simulink model "Com_ISE"  (R2016a)
settings: Solver=VariableStepAuto  StartTime=0.0  StopTime=120  RelTol=1e-3
libraries: simulink x4
settings Model: Creator=Admin  LastModifiedBy=Admin

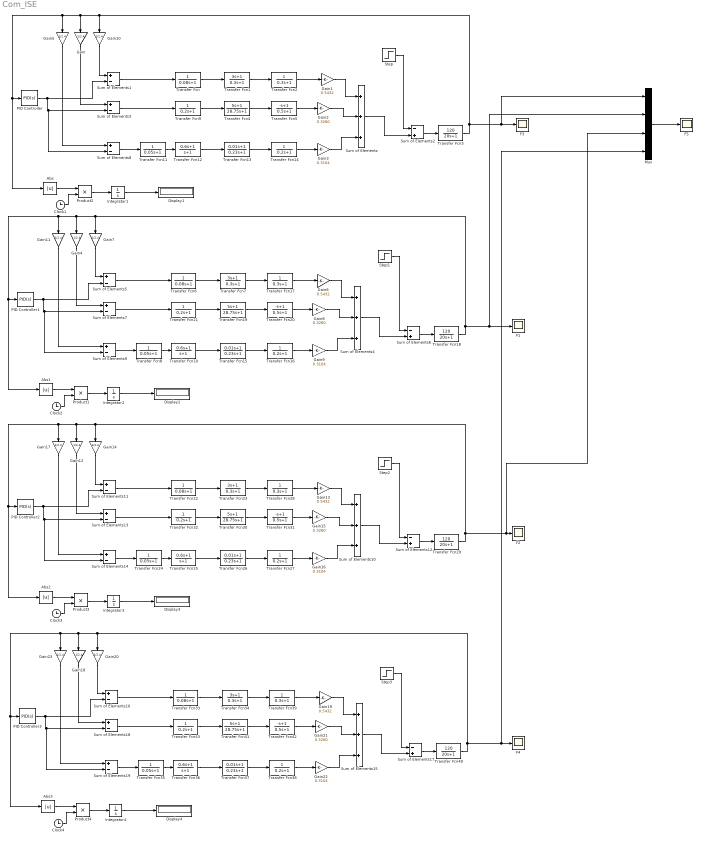
== system Com_ISE ==
  Abs{,1..3} (4 alike) : Abs
  Clock{1..4} (4 alike) : Clock
  Display{1..4} (4 alike) : Display
  F{1..5} (5 alike) : Scope
  Gain{,4..5,7,10..12,14,17..18,20,23} (12 alike) : Gain  Gain=1/2.4
  Gain{1,6,13,19} (4 alike) : Gain  Gain=0.5432
  Gain{2,8,15,21} (4 alike) : Gain  Gain=0.3260
  Gain{3,9,16,22} (4 alike) : Gain  Gain=0.3104
  Integrator{1..4} (4 alike) : Integrator
  Mux : Mux
  PID Controller : simulink/Continuous/PID Controller  Controller=PID  TimeDomain=Continuous-time  SampleTime=-1  IntegratorMethod=Forward Euler  FilterMethod=Forward Euler  Form=Parallel  UseFilter=on  ControllerParametersSource=internal  P=1.2  I=0.4  D=0.11  N=100  InitialConditionSource=internal  InitialConditionForIntegrator=0  InitialConditionForFilter=0  ExternalReset=none  LimitOutput=off  UpperSaturationLimit=inf  LowerSaturationLimit=-inf  LinearizeAsGain=on  AntiWindupMode=none  Kb=1  TrackingMode=off  Kt=1  PParamMin=[]  PParamMax=[]  IParamMin=[]  IParamMax=[]  DParamMin=[]  DParamMax=[]  NParamMin=[]  NParamMax=[]  KbParamMin=[]  KbParamMax=[]  KtParamMin=[]  KtParamMax=[]  POutMin=[]  POutMax=[]  IOutMin=[]  IOutMax=[]  DOutMin=[]  DOutMax=[]  NOutMin=[]  NOutMax=[]  KbOutMin=[]  KbOutMax=[]  KtOutMin=[]  KtOutMax=[]  IntegratorOutMin=[]  IntegratorOutMax=[]  FilterOutMin=[]  FilterOutMax=[]  SumOutMin=[]  SumOutMax=[]  SumI1OutMin=[]  SumI1OutMax=[]  SumI2OutMin=[]  SumI2OutMax=[]  SumI3OutMin=[]  SumI3OutMax=[]  SumDOutMin=[]  SumDOutMax=[]  SaturationOutMin=[]  SaturationOutMax=[]  IntegratorContinuousStateAttributes=''  IntegratorStateMustResolveToSignalObject=off  IntegratorRTWStateStorageClass=Auto  FilterContinuousStateAttributes=''  FilterStateMustResolveToSignalObject=off  FilterRTWStateStorageClass=Auto  DifferentiatorICPrevScaledInput=0  DifferentiatorOutMin=[]  DifferentiatorOutMax=[]
  PID Controller1 : simulink/Continuous/PID Controller  Controller=PID  TimeDomain=Continuous-time  SampleTime=-1  IntegratorMethod=Forward Euler  FilterMethod=Forward Euler  Form=Parallel  UseFilter=on  ControllerParametersSource=internal  P=0.985192773  I=0.993117653  D=0.130440892  N=100  InitialConditionSource=internal  InitialConditionForIntegrator=0  InitialConditionForFilter=0  ExternalReset=none  LimitOutput=off  UpperSaturationLimit=inf  LowerSaturationLimit=-inf  LinearizeAsGain=on  AntiWindupMode=none  Kb=1  TrackingMode=off  Kt=1  PParamMin=[]  PParamMax=[]  IParamMin=[]  IParamMax=[]  DParamMin=[]  DParamMax=[]  NParamMin=[]  NParamMax=[]  KbParamMin=[]  KbParamMax=[]  KtParamMin=[]  KtParamMax=[]  POutMin=[]  POutMax=[]  IOutMin=[]  IOutMax=[]  DOutMin=[]  DOutMax=[]  NOutMin=[]  NOutMax=[]  KbOutMin=[]  KbOutMax=[]  KtOutMin=[]  KtOutMax=[]  IntegratorOutMin=[]  IntegratorOutMax=[]  FilterOutMin=[]  FilterOutMax=[]  SumOutMin=[]  SumOutMax=[]  SumI1OutMin=[]  SumI1OutMax=[]  SumI2OutMin=[]  SumI2OutMax=[]  SumI3OutMin=[]  SumI3OutMax=[]  SumDOutMin=[]  SumDOutMax=[]  SaturationOutMin=[]  SaturationOutMax=[]  IntegratorContinuousStateAttributes=''  IntegratorStateMustResolveToSignalObject=off  IntegratorRTWStateStorageClass=Auto  FilterContinuousStateAttributes=''  FilterStateMustResolveToSignalObject=off  FilterRTWStateStorageClass=Auto  DifferentiatorICPrevScaledInput=0  DifferentiatorOutMin=[]  DifferentiatorOutMax=[]
  PID Controller2 : simulink/Continuous/PID Controller  Controller=PID  TimeDomain=Continuous-time  SampleTime=-1  IntegratorMethod=Forward Euler  FilterMethod=Forward Euler  Form=Parallel  UseFilter=on  ControllerParametersSource=internal  P=0.9999  I=0.9999  D=0.170426245  N=100  InitialConditionSource=internal  InitialConditionForIntegrator=0  InitialConditionForFilter=0  ExternalReset=none  LimitOutput=off  UpperSaturationLimit=inf  LowerSaturationLimit=-inf  LinearizeAsGain=on  AntiWindupMode=none  Kb=1  TrackingMode=off  Kt=1  PParamMin=[]  PParamMax=[]  IParamMin=[]  IParamMax=[]  DParamMin=[]  DParamMax=[]  NParamMin=[]  NParamMax=[]  KbParamMin=[]  KbParamMax=[]  KtParamMin=[]  KtParamMax=[]  POutMin=[]  POutMax=[]  IOutMin=[]  IOutMax=[]  DOutMin=[]  DOutMax=[]  NOutMin=[]  NOutMax=[]  KbOutMin=[]  KbOutMax=[]  KtOutMin=[]  KtOutMax=[]  IntegratorOutMin=[]  IntegratorOutMax=[]  FilterOutMin=[]  FilterOutMax=[]  SumOutMin=[]  SumOutMax=[]  SumI1OutMin=[]  SumI1OutMax=[]  SumI2OutMin=[]  SumI2OutMax=[]  SumI3OutMin=[]  SumI3OutMax=[]  SumDOutMin=[]  SumDOutMax=[]  SaturationOutMin=[]  SaturationOutMax=[]  IntegratorContinuousStateAttributes=''  IntegratorStateMustResolveToSignalObject=off  IntegratorRTWStateStorageClass=Auto  FilterContinuousStateAttributes=''  FilterStateMustResolveToSignalObject=off  FilterRTWStateStorageClass=Auto  DifferentiatorICPrevScaledInput=0  DifferentiatorOutMin=[]  DifferentiatorOutMax=[]
  PID Controller3 : simulink/Continuous/PID Controller  Controller=PID  TimeDomain=Continuous-time  SampleTime=-1  IntegratorMethod=Forward Euler  FilterMethod=Forward Euler  Form=Parallel  UseFilter=on  ControllerParametersSource=internal  P=0.996752419  I=0.999717196  D=0.131550881  N=100  InitialConditionSource=internal  InitialConditionForIntegrator=0  InitialConditionForFilter=0  ExternalReset=none  LimitOutput=off  UpperSaturationLimit=inf  LowerSaturationLimit=-inf  LinearizeAsGain=on  AntiWindupMode=none  Kb=1  TrackingMode=off  Kt=1  PParamMin=[]  PParamMax=[]  IParamMin=[]  IParamMax=[]  DParamMin=[]  DParamMax=[]  NParamMin=[]  NParamMax=[]  KbParamMin=[]  KbParamMax=[]  KtParamMin=[]  KtParamMax=[]  POutMin=[]  POutMax=[]  IOutMin=[]  IOutMax=[]  DOutMin=[]  DOutMax=[]  NOutMin=[]  NOutMax=[]  KbOutMin=[]  KbOutMax=[]  KtOutMin=[]  KtOutMax=[]  IntegratorOutMin=[]  IntegratorOutMax=[]  FilterOutMin=[]  FilterOutMax=[]  SumOutMin=[]  SumOutMax=[]  SumI1OutMin=[]  SumI1OutMax=[]  SumI2OutMin=[]  SumI2OutMax=[]  SumI3OutMin=[]  SumI3OutMax=[]  SumDOutMin=[]  SumDOutMax=[]  SaturationOutMin=[]  SaturationOutMax=[]  IntegratorContinuousStateAttributes=''  IntegratorStateMustResolveToSignalObject=off  IntegratorRTWStateStorageClass=Auto  FilterContinuousStateAttributes=''  FilterStateMustResolveToSignalObject=off  FilterRTWStateStorageClass=Auto  DifferentiatorICPrevScaledInput=0  DifferentiatorOutMin=[]  DifferentiatorOutMax=[]
  Product{1..4} (4 alike) : Product  RndMeth=Zero
  Step{,1..3} (4 alike) : Step  After=0.01  SampleTime=0
  Sum of Elements{,4,10,15} (4 alike) : Sum  Inputs=+++
  Sum of Elements{1,3,5,7..9,11,13..14,16,18..19} (12 alike) : Sum  Inputs=+-
  Sum of Elements{2,6,12,17} (4 alike) : Sum  Inputs=-+
  Transfer Fcn{,6,22,33} (4 alike) : TransferFcn  Denominator=[0.08 1]
  Transfer Fcn{1,7,23,34} (4 alike) : TransferFcn  Numerator=[3 1]  Denominator=[0.3 1]
  Transfer Fcn{10,12,25,36} (4 alike) : TransferFcn  Numerator=[0.6 1]  Denominator=[1 1]
  Transfer Fcn{8,11,24,35} (4 alike) : TransferFcn  Denominator=[0.05 1]
  Transfer Fcn{13,15,26,37} (4 alike) : TransferFcn  Numerator=[0.01 1]  Denominator=[0.23 1]
  Transfer Fcn{9,14,16,21,27,32,38,43} (8 alike) : TransferFcn  Denominator=[0.2 1]
  Transfer Fcn{2,17,28,39} (4 alike) : TransferFcn  Numerator=[ 1]  Denominator=[0.3 1]
  Transfer Fcn{3,18,29,40} (4 alike) : TransferFcn  Numerator=[120]  Denominator=[20 1]
  Transfer Fcn{4,19,30,41} (4 alike) : TransferFcn  Numerator=[5 1]  Denominator=[28.75 1]
  Transfer Fcn{5,20,31,42} (4 alike) : TransferFcn  Numerator=[-1 1]  Denominator=[0.5 1]
  wires:
  Sum of Elements8/1 -> Transfer Fcn11/1
  Transfer Fcn11/1 -> Transfer Fcn12/1
  Transfer Fcn12/1 -> Transfer Fcn13/1
  Transfer Fcn13/1 -> Transfer Fcn14/1
  Transfer Fcn/1 -> Transfer Fcn1/1
  Transfer Fcn1/1 -> Transfer Fcn2/1
  Sum of Elements1/1 -> Transfer Fcn/1
  Transfer Fcn2/1 -> Gain1/1
  Gain1/1 -> Sum of Elements/1
  Sum of Elements3/1 -> Transfer Fcn9/1
  Transfer Fcn9/1 -> Transfer Fcn4/1
  Transfer Fcn4/1 -> Transfer Fcn5/1
  Transfer Fcn5/1 -> Gain2/1
  Gain2/1 -> Sum of Elements/2
  Gain3/1 -> Sum of Elements/3
  Transfer Fcn14/1 -> Gain3/1
  Step/1 -> Sum of Elements2/1
  Sum of Elements/1 -> Sum of Elements2/2
  Sum of Elements2/1 -> Transfer Fcn3/1
  Gain10/1 -> Sum of Elements1/1
  Gain/1 -> Sum of Elements3/1
  Gain5/1 -> Sum of Elements8/1
  Transfer Fcn3/1 -> Mux/1, F3/1, Gain10/1, Gain/1, Gain5/1, Abs/1, PID Controller/1
  PID Controller/1 -> Sum of Elements8/2, Sum of Elements3/2, Sum of Elements1/2
  Abs/1 -> Product2/1
  Clock1/1 -> Product2/2
  Product2/1 -> Integrator1/1
  Integrator1/1 -> Display1/1
  Sum of Elements9/1 -> Transfer Fcn8/1
  Transfer Fcn8/1 -> Transfer Fcn10/1
  Transfer Fcn10/1 -> Transfer Fcn15/1
  Transfer Fcn15/1 -> Transfer Fcn16/1
  Transfer Fcn6/1 -> Transfer Fcn7/1
  Transfer Fcn7/1 -> Transfer Fcn17/1
  Sum of Elements5/1 -> Transfer Fcn6/1
  Transfer Fcn17/1 -> Gain6/1
  Gain6/1 -> Sum of Elements4/1
  Sum of Elements7/1 -> Transfer Fcn21/1
  Transfer Fcn21/1 -> Transfer Fcn19/1
  Transfer Fcn19/1 -> Transfer Fcn20/1
  Transfer Fcn20/1 -> Gain8/1
  Gain8/1 -> Sum of Elements4/2
  Gain9/1 -> Sum of Elements4/3
  Transfer Fcn16/1 -> Gain9/1
  Step1/1 -> Sum of Elements6/1
  Sum of Elements4/1 -> Sum of Elements6/2
  Sum of Elements6/1 -> Transfer Fcn18/1
  Gain7/1 -> Sum of Elements5/1
  Gain4/1 -> Sum of Elements7/1
  Gain11/1 -> Sum of Elements9/1
  PID Controller1/1 -> Sum of Elements9/2, Sum of Elements7/2, Sum of Elements5/2
  Abs1/1 -> Product1/1
  Clock2/1 -> Product1/2
  Product1/1 -> Integrator2/1
  Integrator2/1 -> Display2/1
  Sum of Elements14/1 -> Transfer Fcn24/1
  Transfer Fcn24/1 -> Transfer Fcn25/1
  Transfer Fcn25/1 -> Transfer Fcn26/1
  Transfer Fcn26/1 -> Transfer Fcn27/1
  Transfer Fcn22/1 -> Transfer Fcn23/1
  Transfer Fcn23/1 -> Transfer Fcn28/1
  Sum of Elements11/1 -> Transfer Fcn22/1
  Transfer Fcn28/1 -> Gain13/1
  Gain13/1 -> Sum of Elements10/1
  Sum of Elements13/1 -> Transfer Fcn32/1
  Transfer Fcn32/1 -> Transfer Fcn30/1
  Transfer Fcn30/1 -> Transfer Fcn31/1
  Transfer Fcn31/1 -> Gain15/1
  Gain15/1 -> Sum of Elements10/2
  Gain16/1 -> Sum of Elements10/3
  Transfer Fcn27/1 -> Gain16/1
  Step2/1 -> Sum of Elements12/1
  Sum of Elements10/1 -> Sum of Elements12/2
  Sum of Elements12/1 -> Transfer Fcn29/1
  Gain14/1 -> Sum of Elements11/1
  Gain12/1 -> Sum of Elements13/1
  Gain17/1 -> Sum of Elements14/1
  PID Controller2/1 -> Sum of Elements14/2, Sum of Elements13/2, Sum of Elements11/2
  Abs2/1 -> Product3/1
  Clock3/1 -> Product3/2
  Product3/1 -> Integrator3/1
  Integrator3/1 -> Display3/1
  Sum of Elements19/1 -> Transfer Fcn35/1
  Transfer Fcn35/1 -> Transfer Fcn36/1
  Transfer Fcn36/1 -> Transfer Fcn37/1
  Transfer Fcn37/1 -> Transfer Fcn38/1
  Transfer Fcn33/1 -> Transfer Fcn34/1
  Transfer Fcn34/1 -> Transfer Fcn39/1
  Sum of Elements16/1 -> Transfer Fcn33/1
  Transfer Fcn39/1 -> Gain19/1
  Gain19/1 -> Sum of Elements15/1
  Sum of Elements18/1 -> Transfer Fcn43/1
  Transfer Fcn43/1 -> Transfer Fcn41/1
  Transfer Fcn41/1 -> Transfer Fcn42/1
  Transfer Fcn42/1 -> Gain21/1
  Gain21/1 -> Sum of Elements15/2
  Gain22/1 -> Sum of Elements15/3
  Transfer Fcn38/1 -> Gain22/1
  Step3/1 -> Sum of Elements17/1
  Sum of Elements15/1 -> Sum of Elements17/2
  Sum of Elements17/1 -> Transfer Fcn40/1
  Gain20/1 -> Sum of Elements16/1
  Gain18/1 -> Sum of Elements18/1
  Gain23/1 -> Sum of Elements19/1
  Transfer Fcn40/1 -> Mux/4, F4/1, Gain20/1, Gain18/1, Gain23/1, Abs3/1, PID Controller3/1
  PID Controller3/1 -> Sum of Elements19/2, Sum of Elements18/2, Sum of Elements16/2
  Abs3/1 -> Product4/1
  Clock4/1 -> Product4/2
  Product4/1 -> Integrator4/1
  Integrator4/1 -> Display4/1
  Mux/1 -> F5/1
  Transfer Fcn18/1 -> Mux/2, F1/1, Gain7/1, Gain4/1, Gain11/1, Abs1/1, PID Controller1/1
  Transfer Fcn29/1 -> Mux/3, F2/1, Gain14/1, Gain12/1, Gain17/1, Abs2/1, PID Controller2/1
